simulink library "abdopulkader_library"  (R2017b)
settings: Solver=VariableStepAuto  StartTime=0.0  StopTime=10.0  RelTol=1e-3
settings Model: Creator=abdoul kader  LastModifiedBy=abdoul kader

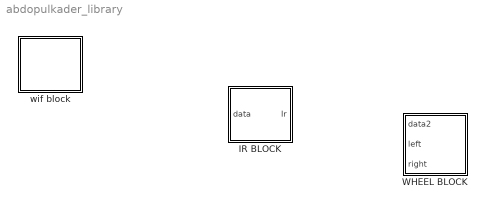
== system abdopulkader_library ==
  IR BLOCK : Stateflow chart  TreatAsAtomicUnit=on
  WHEEL BLOCK : Stateflow chart  TreatAsAtomicUnit=on
  wif block : Stateflow chart  TreatAsAtomicUnit=on

== stateflow chart abdopulkader_library/IR BLOCK ==
  state tf
    en,du:
    Ir=IRA;
  data: Ir output; data input
  function IR:
    | function IR
    | y=[0,0,0,0,0,0,];
    | persistent obj
    | coder.extrinsic('evalin');
    | coder.extrinsic('get');
    | if isempty(obj)
    |     obj=evalin('base','re');
    | end
    | coder.extrinsic('RangeStateRoomba');
    | y=RangeStateRoomba(obj);

== stateflow chart abdopulkader_library/WHEEL BLOCK ==
  state kader
    entry,during:
    motor(right,left)
  data: data2 input; left input; right input
  function motor:
    | function motor
    | persistent obj
    | coder.extrinsic('RoomBaWiFi')
    | coder.extrinsic('assignin');
    | if isempty(obj)
    |     obj=RoomBaWiFi('10.0.0.1','full')
    | end
    | assignin('base','re',obj)

== stateflow chart abdopulkader_library/wif block ==
  state b
    entry,during:
    wifi;
    op=0;
  function wifi:
    | function wifi
    | persistent obj
    | coder.extrinsic('RoomBaWiFi')
    | coder.extrinsic('assignin');
    | if isempty(obj)
    |     obj=RoomBaWiFi('10.0.0.1','full')
    | end
    | assignin('base','re',obj)
